simulink model "S3"  (R2023b)
settings: Solver=FixedStepAuto  StartTime=0.0  StopTime=10  FixedStep=Step_T  RelTol=1e-3
values from neighbouring files (symbols this model uses):
  seed = 9531    [P_sim.m]
  Step_T = 0.001    [P_sim.m]
  x_1_0 = 1    [P_sim.m]
  x_2_0 = -2    [P_sim.m]
undefined symbols (not defined in the file or in its folder): alpha_1_d_0, pam
settings Model: Creator=admin  LastModifiedBy=admin

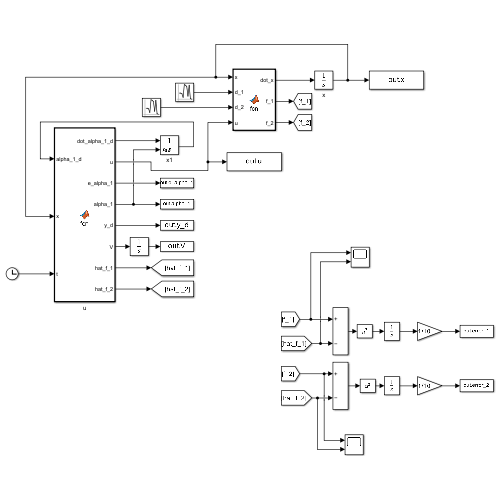
[thumbnail: Simulink's stored preview of the top-level diagram]
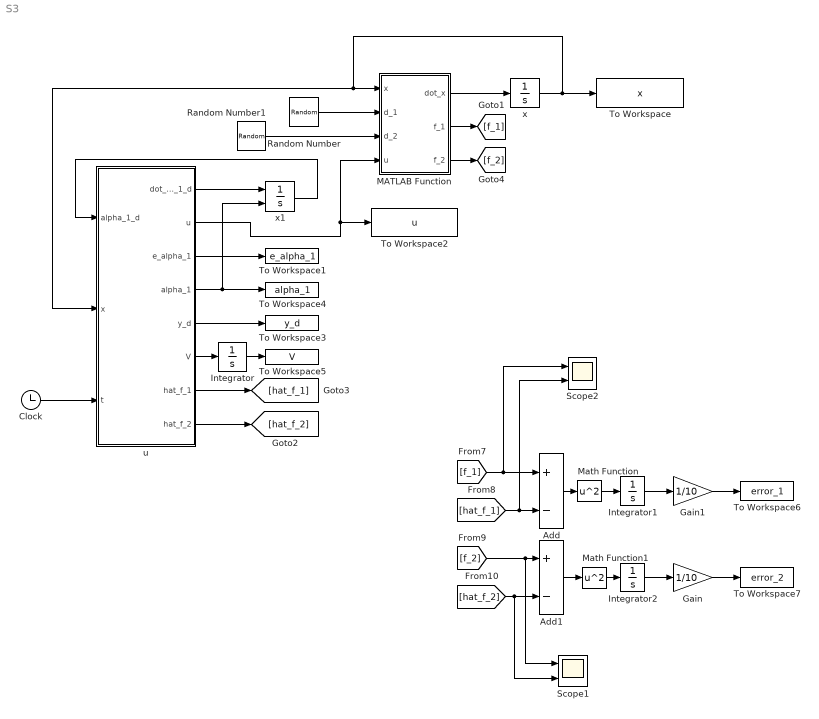
== system S3 ==
  Add : Sum  Inputs=+-
  Add1 : Sum  Inputs=+-
  Clock : Clock
  Gain : Gain  Gain=1/10
  Gain1 : Gain  Gain=1/10
  Integrator : Integrator
  Integrator1 : Integrator
  Integrator2 : Integrator
  MATLAB Function : MATLAB Function  TreatAsAtomicUnit=on
  Math Function : Math  Operator=square
  Math Function1 : Math  Operator=square
  Random Number : RandomNumber  Variance=pam.d*pam.d  Seed=-seed  SampleTime=Step_T
  Random Number1 : RandomNumber  Variance=pam.d*pam.d  Seed=seed  SampleTime=Step_T
  Scope1 : Scope  NumInputPorts=2
  Scope2 : Scope  NumInputPorts=2
  To Workspace : ToWorkspace  VariableName=x  SaveFormat=Timeseries  SampleTime=-1
  To Workspace1 : ToWorkspace  VariableName=e_alpha_1  SaveFormat=Timeseries  SampleTime=-1
  To Workspace2 : ToWorkspace  VariableName=u  SaveFormat=Timeseries  SampleTime=-1
  To Workspace3 : ToWorkspace  VariableName=y_d  SaveFormat=Timeseries  SampleTime=-1
  To Workspace4 : ToWorkspace  VariableName=alpha_1  SaveFormat=Timeseries  SampleTime=-1
  To Workspace5 : ToWorkspace  VariableName=V  SaveFormat=Timeseries  SampleTime=-1
  To Workspace6 : ToWorkspace  VariableName=error_1  SaveFormat=Timeseries  SampleTime=-1
  To Workspace7 : ToWorkspace  VariableName=error_2  SaveFormat=Timeseries  SampleTime=-1
  u : MATLAB Function  TreatAsAtomicUnit=on
  x : Integrator  InitialCondition=[x_1_0;x_2_0]
  x1 : Integrator  InitialConditionSource=external  InitialCondition=alpha_1_d_0
  wires:
  MATLAB Function/1(dot_x) -> x/1
  x/1 -> u/2(x), MATLAB Function/1(x), To Workspace/1
  u/2(u) -> MATLAB Function/4(u), To Workspace2/1
  u/3(e_alpha_1) -> To Workspace1/1
  u/5(y_d) -> To Workspace3/1
  Clock/1 -> u/3(t)
  u/1(dot_alpha_1_d) -> x1/1
  x1/1 -> u/1(alpha_1_d)
  u/4(alpha_1) -> x1/2, To Workspace4/1
  u/6(V) -> Integrator/1
  Integrator/1 -> To Workspace5/1
  Random Number/1 -> MATLAB Function/2(d_1)
  Random Number1/1 -> MATLAB Function/3(d_2)
  Gain1/1 -> To Workspace6/1
  Math Function1/1 -> Integrator2/1
  Gain/1 -> To Workspace7/1
  Math Function/1 -> Integrator1/1
  [hat_f_2] -> Scope1/2, Add1/2
  Integrator2/1 -> Gain/1
  Add/1 -> Math Function/1
  [hat_f_1] -> Scope2/2, Add/2
  [f_1] -> Scope2/1, Add/1
  Add1/1 -> Math Function1/1
  [f_2] -> Scope1/1, Add1/1
  Integrator1/1 -> Gain1/1
  MATLAB Function/3(f_2) -> [f_2]
  MATLAB Function/2(f_1) -> [f_1]
  u/8(hat_f_2) -> [hat_f_2]
  u/7(hat_f_1) -> [hat_f_1]

== matlab function S3/u ==
  data: alpha_1_d input; dot_alpha_1_d output; x input; t input; u output; e_alpha_1 output; alpha_1 output; pam parameter; y_d output; V output; hat_f_1 output; hat_f_2 output
function [dot_alpha_1_d,u,e_alpha_1,alpha_1,y_d,V,hat_f_1,hat_f_2]  = fcn(alpha_1_d,x,t,pam)

y_d = 0;
dot_y_d = 0;

x_1 = x(1);
x_2 = x(2);

z_1 = [x_1;cos(x_1)];
z_2 = [x_1;x_2;sin(x_1)*cos(x_2)];

%% 第一阶
e_1 = x_1 - y_d;
alpha_1 = -pam.lambda_1*e_1-pam.hat_theta_1'*z_1+dot_y_d;

%% 第二阶
e_2 = x_2 - alpha_1;
dot_alpha_1_d = -(1/pam.omega_1)*(alpha_1_d-alpha_1);
u = -pam.lambda_2*e_2-pam.hat_theta_2'*z_2+dot_alpha_1_d;
e_alpha_1 = alpha_1_d-alpha_1;

V = e_1^2+u^2;

hat_f_1=pam.hat_theta_1'*z_1;
hat_f_2=pam.hat_theta_2'*z_2;

== matlab function S3/MATLAB Function ==
  data: x input; d_1 input; d_2 input; dot_x output; u input; pam parameter; f_1 output; f_2 output
function [dot_x,f_1,f_2]  = fcn(x,d_1,d_2,u,pam)

x_1 = x(1);
x_2 = x(2);

dot_x_1 = x_2-(1/pam.beta_1-pam.rho_1+sqrt(2))*x_1+cos(x_1)+d_1;
dot_x_2 = u+sqrt(5)*x_1-(1/pam.beta_2-pam.rho_2)*x_2+sqrt(2)*sin(x_1)*cos(x_2)+d_2;

dot_x = [dot_x_1;dot_x_2];
f_1 = -(1/pam.beta_1-pam.rho_1+sqrt(2))*x_1+cos(x_1);
f_2 = sqrt(5)*x_1-(1/pam.beta_2-pam.rho_2)*x_2+sqrt(2)*sin(x_1)*cos(x_2);
